simulink model "Controller_with_3DOF_model"  (R2020a)
settings: Solver=ode4  StartTime=0.0  StopTime=130  FixedStep=0.04  RelTol=1e-3
values from neighbouring files (symbols this model uses):
  a = L*(1-WF)    (= 1.81178)    [parameters.m]
  avg_dist = mean(dist_array)    [parameters.m]
  b = L*WF    (= 1.32822)    [parameters.m]
  c2r = 1*(pi/180)    (= 0.0174532925199)    [parameters.m]
  m = 2257    [parameters.m]
  n = 12    [parameters.m]
  X_waypoints = [699934.396313 699934.399288 699934.40266 699934.406729 699934.412322 699934.420718 699934.432825 699934.447764 699934.466045 699934.489064 699934.518829 699934.556022 ... (1891 elements, 1x1891)]    [reference_path.mat]
  Y_waypoints = [-5195211.87 -5195211.87121 -5195211.87256 -5195211.87411 -5195211.87621 -5195211.87926 -5195211.88371 -5195211.88919 -5195211.8959 -5195211.90452 -5195211.91606 -5195211.93042 ... (1891 elements, 1x1891)]    [reference_path.mat]
  Yaw_waypoint = [130.3891316 130.393107092 130.397831164 130.402362614 130.409271739 130.418915142 130.433687561 130.450949982 130.469948658 130.492496199 130.52263774 130.556853638 ... (1891 elements, 1x1891)]    [reference_path.mat]
undefined symbols (not defined in the file or in its folder): C_alpha, Kp_crosstrack, Kp_yaw, Kp_yaw_rate, mass
libraries: simulink_extras x11, simulink x3, autolibshared x1
settings Model: Creator=bhagwat  LastModifiedBy=root

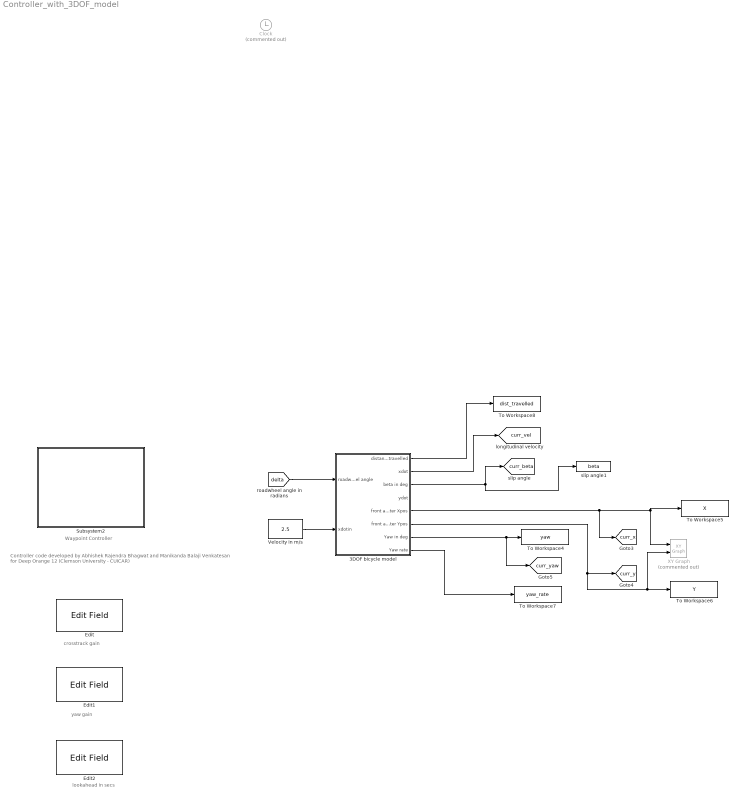
== system Controller_with_3DOF_model ==
  note: Controller code developed by Abhishek Rajendra Bhagwat and
      | Manikanda Balaji Venkatesan for Deep Orange 12 (Clemson University - CUICAR)
  note: crosstrack gain
  note: Waypoint Controller
  note: yaw gain
  note: lookahead in secs
  3DOF bicycle model : Subsystem
  Clock : Clock  Commented=on
  Edit : EditField  LabelPosition=Hide  ShowInitialText=on  Alignment=Center
  Edit1 : EditField  LabelPosition=Hide  ShowInitialText=on  Alignment=Center
  Edit2 : EditField  LabelPosition=Hide  ShowInitialText=on  Alignment=Center
  Subsystem2 : Subsystem
  To Workspace4 : ToWorkspace  VariableName=yaw  SaveFormat=Timeseries  SampleTime=-1
  To Workspace5 : ToWorkspace  VariableName=X  SampleTime=-1
  To Workspace6 : ToWorkspace  VariableName=Y  SampleTime=-1
  To Workspace7 : ToWorkspace  VariableName=yaw_rate  SaveFormat=Timeseries  SampleTime=-1
  To Workspace8 : ToWorkspace  VariableName=dist_travelled  SaveFormat=Timeseries  SampleTime=-1
  Velocity in m/s : Constant  Value=2.5
  XY Graph : simulink/Sinks/XY Graph  Commented=on  xmin=-1000  xmax=1000  ymin=-1000  ymax=1000  st=-1
  slip angle1 : ToWorkspace  VariableName=beta  SaveFormat=Timeseries  SampleTime=-1
  tag scope: curr_beta=global, curr_vel=global, curr_x=global, curr_y=global, curr_yaw=global
  wires:
  3DOF bicycle model/7(Yaw in deg) -> [curr_yaw], To Workspace4/1
  3DOF bicycle model/3(beta in deg) -> [curr_beta], slip angle1/1
  3DOF bicycle model/6(front axle center Ypos) -> XY Graph/2, To Workspace6/1, [curr_y]
  3DOF bicycle model/5(front axle center Xpos) -> To Workspace5/1, XY Graph/1, [curr_x]
  [delta] -> 3DOF bicycle model/1(roadwheel angle)
  Velocity in m/s/1 -> 3DOF bicycle model/2(xdotin)
  3DOF bicycle model/1(distance travelled) -> To Workspace8/1
  3DOF bicycle model/2(xdot) -> [curr_vel]
  3DOF bicycle model/8(Yaw rate) -> To Workspace7/1

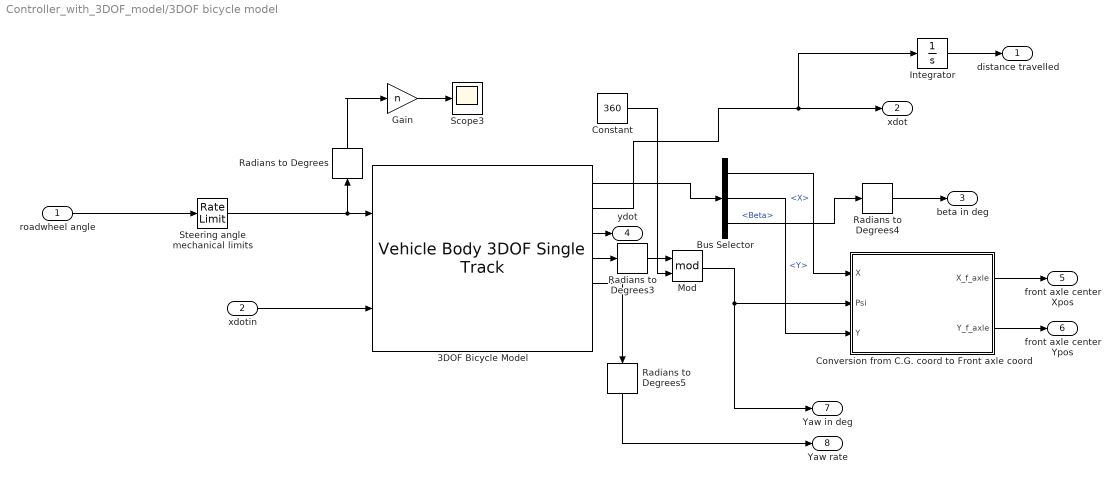
== system Controller_with_3DOF_model/3DOF bicycle model ==
  roadwheel angle : Inport
  xdotin : Inport  Port=2
  3DOF Bicycle Model : autolibshared/Vehicle Body 3DOF Single Track  trackMode=Single (bicycle)  inputMode=External longitudinal velocity  frontSteerMode=on  rearSteerMode=off  windMode=off  muMode=off  extFMode=off  extMMode=off  extXo=off  extpsio=off  extxdoto=off  extro=off  extYo=off  extTamb=off  extydoto=off  aMode=2  NF=2  NR=2  m=m  a=a  b=b  h=0.35  X_o=X_waypoints(1)  xdot_o=0  CalphaMode=off  sigmaMode=off  d=0  w=[1.4,1.4]  Cy_f=C1_0  Cy_r=C2_0  sigma_f=.1  sigma_r=.1  alpha_f_brk=[-.1 .1]  Cy_f_data=[-9e3 9e3]  alpha_r_brk=[-.1 .1]  Cy_r_data=[-9e3 9e3]  Y_o=Y_waypoints(1)  ydot_o=0  Izz=2500  psi_o=(360+100-Yaw_waypoint(1))*c2r  r_o=0  Af=2  Cd=.3  Cl=.1  Cpm=.1  beta_w=[0:0.01:0.3]  Cs=[0:0.03:0.9]  Cym=[0:0.01:0.3]  Pabs=101325  Tair=273  g=9.81  mu=1  xdot_tol=.01  Fznom=5000  Fxtire_sat=7e4  Fytire_sat=7e4  longOff=0  latOff=0  vertOff=0  wrapAng=off
      settings: SourceProductBaseCode=PW,MT,VE,VP
  Bus Selector : BusSelector  OutputSignals=InertFrm.Cg.Disp.X,InertFrm.Cg.Disp.Y,BdyFrm.Cg.Ang.Beta
  Constant : Constant  Value=360
  Conversion from C.G. coord to Front axle coord : Subsystem
  Gain : Gain  Gain=n
  Integrator : Integrator
  Mod : Math  Operator=mod  SaturateOnIntegerOverflow=on
  Radians to Degrees{,3..5} (4 alike) : simulink_extras/Transformations/Radians to Degrees
  Scope3 : Scope
  Steering angle mechanical limits : RateLimiter  RisingSlewLimit=275/n  FallingSlewLimit=-275/n  SampleTimeMode=inherited
  distance travelled : Outport
  xdot : Outport  Port=2
  beta in deg : Outport  Port=3
  ydot : Outport  Port=4
  front axle center Xpos : Outport  Port=5
  front axle center Ypos : Outport  Port=6
  Yaw in deg : Outport  Port=7
  Yaw rate : Outport  Port=8
  wires:
  3DOF Bicycle Model/3 -> ydot/1
  Steering angle mechanical limits/1 -> Radians to Degrees/1, 3DOF Bicycle Model/1
  Radians to Degrees5/1 -> Yaw rate/1
  3DOF Bicycle Model/4 -> Radians to Degrees3/1
  3DOF Bicycle Model/2 -> xdot/1, Integrator/1
  3DOF Bicycle Model/1 -> Bus Selector/1
  roadwheel angle/1 -> Steering angle mechanical limits/1
  Radians to Degrees4/1 -> beta in deg/1
  Mod/1 -> Yaw in deg/1, Conversion from C.G. coord to Front axle coord/2(Psi)
  xdotin/1 -> 3DOF Bicycle Model/2
  3DOF Bicycle Model/5 -> Radians to Degrees5/1
  Bus Selector/2 -> Conversion from C.G. coord to Front axle coord/3(Y)  "<Y>"
  Integrator/1 -> distance travelled/1
  Radians to Degrees3/1 -> Mod/1
  Bus Selector/1 -> Conversion from C.G. coord to Front axle coord/1(X)  "<X>"
  Bus Selector/3 -> Radians to Degrees4/1  "<Beta>"
  Radians to Degrees/1 -> Gain/1
  Gain/1 -> Scope3/1
  Conversion from C.G. coord to Front axle coord/2(Y_f_axle) -> front axle center Ypos/1
  Conversion from C.G. coord to Front axle coord/1(X_f_axle) -> front axle center Xpos/1
  Constant/1 -> Mod/2

== system Controller_with_3DOF_model/Subsystem2 ==
  Reference waypoints : Subsystem
  Steering Wheel Angle : Subsystem
  Vehicle state : Subsystem

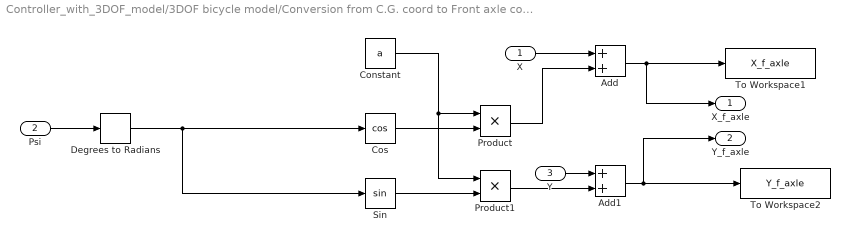
== system Controller_with_3DOF_model/3DOF bicycle model/Conversion from C.G. coord to Front axle coord ==
  X : Inport
  Psi : Inport  Port=2
  Y : Inport  Port=3
  Add : Sum
  Add1 : Sum
  Constant : Constant  Value=a
  Cos : Trigonometry  Operator=cos
  Degrees to Radians : simulink_extras/Transformations/Degrees to Radians
  Product : Product
  Product1 : Product
  Sin : Trigonometry
  To Workspace1 : ToWorkspace  VariableName=X_f_axle  SaveFormat=Timeseries  SampleTime=-1
  To Workspace2 : ToWorkspace  VariableName=Y_f_axle  SaveFormat=Timeseries  SampleTime=-1
  X_f_axle : Outport
  Y_f_axle : Outport  Port=2
  wires:
  Cos/1 -> Product/2
  Sin/1 -> Product1/2
  Product/1 -> Add/2
  Constant/1 -> Product1/1, Product/1
  X/1 -> Add/1
  Add1/1 -> Y_f_axle/1, To Workspace2/1
  Psi/1 -> Degrees to Radians/1
  Add/1 -> To Workspace1/1, X_f_axle/1
  Product1/1 -> Add1/2
  Y/1 -> Add1/1
  Degrees to Radians/1 -> Cos/1, Sin/1

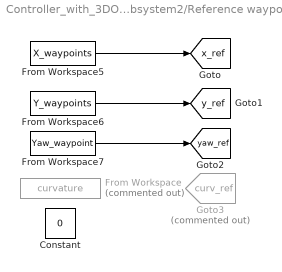
== system Controller_with_3DOF_model/Subsystem2/Reference waypoints ==
  Constant : Constant  Value=0
  From Workspace : FromWorkspace  Commented=on  VariableName=curvature
  From Workspace5 : FromWorkspace  VariableName=X_waypoints
  From Workspace6 : FromWorkspace  VariableName=Y_waypoints
  From Workspace7 : FromWorkspace  VariableName=Yaw_waypoint
  Goto3 : Goto  Commented=on  GotoTag=curv_ref  TagVisibility=global
  tag scope: x_ref=global, y_ref=global, yaw_ref=global
  wires:
  From Workspace5/1 -> [x_ref]
  From Workspace6/1 -> [y_ref]
  From Workspace7/1 -> [yaw_ref]

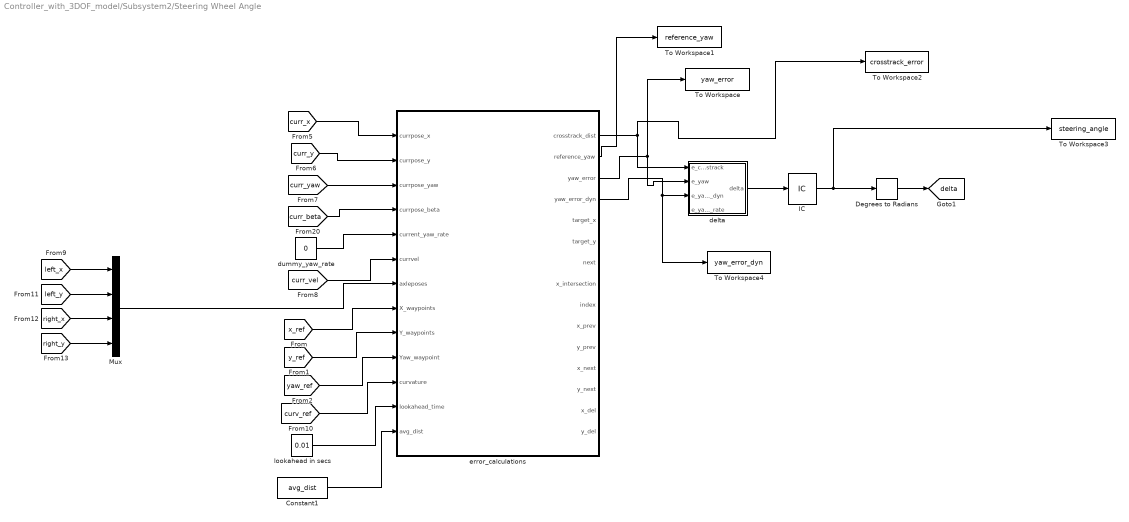
== system Controller_with_3DOF_model/Subsystem2/Steering Wheel Angle ==
  Constant1 : Constant  Value=avg_dist
  Degrees to Radians : simulink_extras/Transformations/Degrees to Radians
  IC : InitialCondition  Value=0
  Mux : Mux
  To Workspace : ToWorkspace  VariableName=yaw_error  SaveFormat=Timeseries  SampleTime=-1
  To Workspace1 : ToWorkspace  VariableName=reference_yaw  SaveFormat=Timeseries  SampleTime=-1
  To Workspace2 : ToWorkspace  VariableName=crosstrack_error  SaveFormat=Timeseries  SampleTime=-1
  To Workspace3 : ToWorkspace  VariableName=steering_angle  SaveFormat=Timeseries  SampleTime=-1
  To Workspace4 : ToWorkspace  VariableName=yaw_error_dyn  SaveFormat=Timeseries  SampleTime=-1
  delta : Subsystem
  dummy_yaw_rate : Constant  Value=0
  error_calculations : MATLAB Function  TreatAsAtomicUnit=on
  lookahead in secs : Constant  Value=0.01
  tag scope: delta=global
  wires:
  [yaw_ref] -> error_calculations/10(Yaw_waypoint)
  [curv_ref] -> error_calculations/11(curvature)
  [x_ref] -> error_calculations/8(X_waypoints)
  [y_ref] -> error_calculations/9(Y_waypoints)
  error_calculations/3(yaw_error) -> delta/2(e_yaw), To Workspace/1
  [curr_x] -> error_calculations/1(currpose_x)
  [curr_y] -> error_calculations/2(currpose_y)
  [curr_yaw] -> error_calculations/3(currpose_yaw)
  dummy_yaw_rate/1 -> error_calculations/5(current_yaw_rate)
  [curr_vel] -> error_calculations/6(currvel)
  Mux/1 -> error_calculations/7(axleposes)
  [left_x] -> Mux/1
  [left_y] -> Mux/2
  [right_x] -> Mux/3
  [right_y] -> Mux/4
  [curr_beta] -> error_calculations/4(currpose_beta)
  error_calculations/2(reference_yaw) -> To Workspace1/1
  Degrees to Radians/1 -> [delta]
  delta/1(delta) -> IC/1
  IC/1 -> To Workspace3/1, Degrees to Radians/1
  error_calculations/4(yaw_error_dyn) -> To Workspace4/1, delta/3(e_yaw_dyn)
  Constant1/1 -> error_calculations/13(avg_dist)
  lookahead in secs/1 -> error_calculations/12(lookahead_time)
  error_calculations/1(crosstrack_dist) -> To Workspace2/1, delta/1(e_crosstrack)

== system Controller_with_3DOF_model/Subsystem2/Vehicle state ==
  left_right_wheel_coordinates : Subsystem
  position : Subsystem  Commented=on

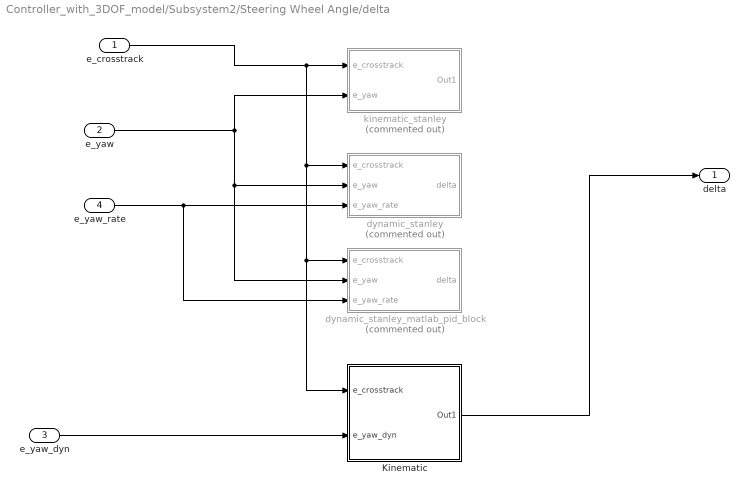
== system Controller_with_3DOF_model/Subsystem2/Steering Wheel Angle/delta ==
  e_crosstrack : Inport
  e_yaw : Inport  Port=2
  e_yaw_dyn : Inport  Port=3
  e_yaw_rate : Inport  Port=4
  Kinematic : Subsystem
  dynamic_stanley : Subsystem  Commented=on
  dynamic_stanley_matlab_pid_block : Subsystem  Commented=on
  kinematic_stanley : Subsystem  Commented=on
  delta : Outport
  wires:
  e_crosstrack/1 -> Kinematic/1(e_crosstrack), dynamic_stanley_matlab_pid_block/1(e_crosstrack), dynamic_stanley/1(e_crosstrack), kinematic_stanley/1(e_crosstrack)
  e_yaw/1 -> dynamic_stanley_matlab_pid_block/2(e_yaw), dynamic_stanley/2(e_yaw), kinematic_stanley/2(e_yaw)
  e_yaw_rate/1 -> dynamic_stanley_matlab_pid_block/3(e_yaw_rate), dynamic_stanley/3(e_yaw_rate)
  Kinematic/1(Out1) -> delta/1
  e_yaw_dyn/1 -> Kinematic/2(e_yaw_dyn)

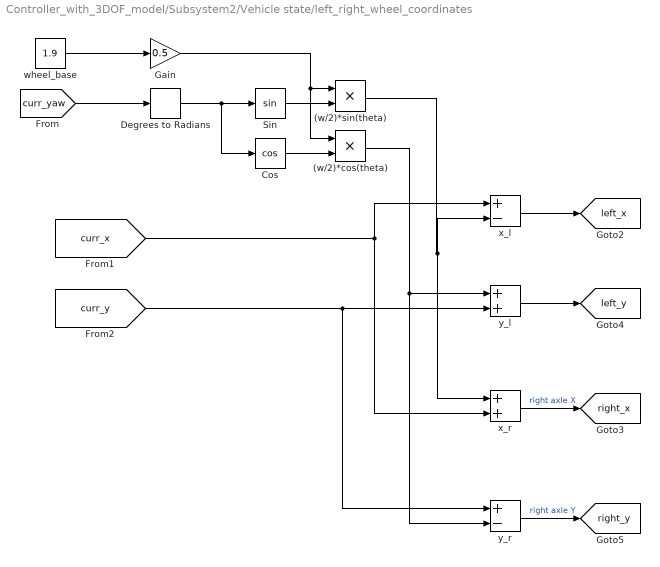
== system Controller_with_3DOF_model/Subsystem2/Vehicle state/left_right_wheel_coordinates ==
  (w/2)*cos(theta) : Product
  (w/2)*sin(theta) : Product
  Cos : Trigonometry  Operator=cos
  Degrees to Radians : simulink_extras/Transformations/Degrees to Radians
  Gain : Gain  Gain=0.5
  Sin : Trigonometry
  wheel_base : Constant  Value=1.9
  x_l : Sum  Inputs=+-
  x_r : Sum
  y_l : Sum
  y_r : Sum  Inputs=+-
  tag scope: left_x=global, left_y=global, right_x=global, right_y=global
  wires:
  wheel_base/1 -> Gain/1
  Degrees to Radians/1 -> Cos/1, Sin/1
  Sin/1 -> (w/2)*sin(theta)/2
  Gain/1 -> (w/2)*cos(theta)/1, (w/2)*sin(theta)/1
  Cos/1 -> (w/2)*cos(theta)/2
  (w/2)*sin(theta)/1 -> x_r/1, x_l/2
  [curr_y] -> y_r/1, y_l/2
  [curr_x] -> x_r/2, x_l/1
  (w/2)*cos(theta)/1 -> y_r/2, y_l/1
  [curr_yaw] -> Degrees to Radians/1
  y_r/1 -> [right_y]  "right axle Y"
  x_r/1 -> [right_x]  "right axle X"
  x_l/1 -> [left_x]
  y_l/1 -> [left_y]

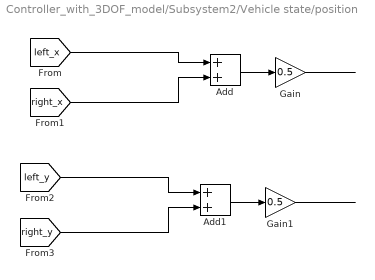
== system Controller_with_3DOF_model/Subsystem2/Vehicle state/position ==
  Add : Sum
  Add1 : Sum
  Gain : Gain  Gain=0.5
  Gain1 : Gain  Gain=0.5
  wires:
  Add/1 -> Gain/1
  Gain1/1 -> ?
  Gain/1 -> ?
  Add1/1 -> Gain1/1
  [left_x] -> Add/1
  [right_x] -> Add/2
  [left_y] -> Add1/1
  [right_y] -> Add1/2

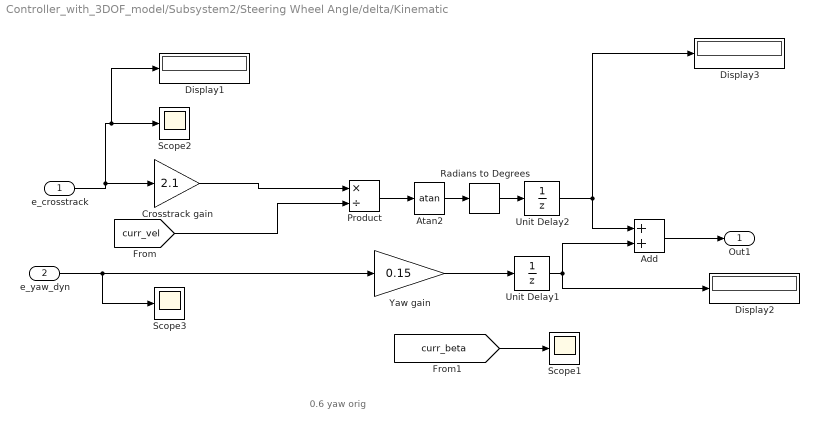
== system Controller_with_3DOF_model/Subsystem2/Steering Wheel Angle/delta/Kinematic ==
  note: 0.6 yaw orig
  e_crosstrack : Inport
  e_yaw_dyn : Inport  Port=2
  Add : Sum
  Atan2 : Trigonometry  Operator=atan  OutputSignalType=real
  Crosstrack gain : Gain  Gain=2.1
  Display1 : Display
  Display2 : Display
  Display3 : Display
  Product : Product  Inputs=*/
  Radians to Degrees : simulink_extras/Transformations/Radians to Degrees
  Scope1 : Scope
  Scope2 : Scope
  Scope3 : Scope
  Unit Delay1 : UnitDelay  SampleTime=-1  HasFrameUpgradeWarning=on
  Unit Delay2 : UnitDelay  SampleTime=-1  HasFrameUpgradeWarning=on
  Yaw gain : Gain  Gain=0.15
  Out1 : Outport
  wires:
  Add/1 -> Out1/1
  [curr_vel] -> Product/2
  Radians to Degrees/1 -> Unit Delay2/1
  Atan2/1 -> Radians to Degrees/1
  Unit Delay1/1 -> Add/2, Display2/1
  e_yaw_dyn/1 -> Scope3/1, Yaw gain/1
  Yaw gain/1 -> Unit Delay1/1
  Crosstrack gain/1 -> Product/1
  Product/1 -> Atan2/1
  e_crosstrack/1 -> Display1/1, Scope2/1, Crosstrack gain/1
  [curr_beta] -> Scope1/1
  Unit Delay2/1 -> Display3/1, Add/1

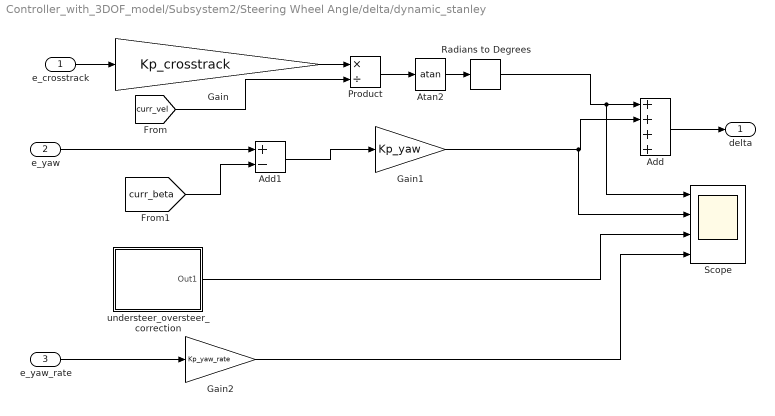
== system Controller_with_3DOF_model/Subsystem2/Steering Wheel Angle/delta/dynamic_stanley ==
  e_crosstrack : Inport
  e_yaw : Inport  Port=2
  e_yaw_rate : Inport  Port=3
  Add : Sum  Inputs=++++
  Add1 : Sum  Inputs=+-
  Atan2 : Trigonometry  Operator=atan  OutputSignalType=real
  Gain : Gain  Gain=Kp_crosstrack
  Gain1 : Gain  Gain=Kp_yaw
  Gain2 : Gain  Gain=Kp_yaw_rate
  Product : Product  Inputs=*/
  Radians to Degrees : simulink_extras/Transformations/Radians to Degrees
  Scope : Scope  NumInputPorts=4
  understeer_oversteer_correction : Subsystem
  delta : Outport
  wires:
  e_crosstrack/1 -> Gain/1
  Product/1 -> Atan2/1
  Gain/1 -> Product/1
  e_yaw/1 -> Add1/1
  Gain1/1 -> Scope/2, Add/2
  Atan2/1 -> Radians to Degrees/1
  Radians to Degrees/1 -> Scope/1, Add/1
  [curr_vel] -> Product/2
  Add/1 -> delta/1
  [curr_beta] -> Add1/2
  Add1/1 -> Gain1/1
  understeer_oversteer_correction/1(Out1) -> Scope/3
  e_yaw_rate/1 -> Gain2/1
  Gain2/1 -> Scope/4

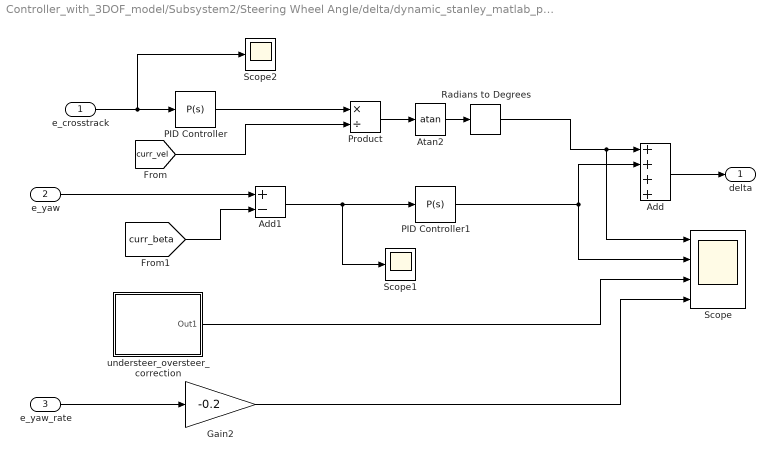
== system Controller_with_3DOF_model/Subsystem2/Steering Wheel Angle/delta/dynamic_stanley_matlab_pid_block ==
  e_crosstrack : Inport
  e_yaw : Inport  Port=2
  e_yaw_rate : Inport  Port=3
  Add : Sum  Inputs=++++
  Add1 : Sum  Inputs=+-
  Atan2 : Trigonometry  Operator=atan  OutputSignalType=real
  Gain2 : Gain  Gain=-0.2
  PID Controller : simulink/Continuous/PID Controller  Controller=P  Form=Parallel  TimeDomain=Continuous-time  UseExternalTs=off  SampleTime=-1  IntegratorMethod=Forward Euler  FilterMethod=Forward Euler  ControllerParametersSource=internal  P=2  I=-1  D=0  UseFilter=on  N=100  TunerSelectOption=Transfer Function Based (PID Tuner App)  InitialConditionSource=internal  InitialConditionForIntegrator=0  InitialConditionForFilter=0  DifferentiatorICPrevScaledInput=0  ExternalReset=none  TrackingMode=off  Kt=1  LimitOutput=off  UpperSaturationLimit=inf  LowerSaturationLimit=-inf  LinearizeAsGain=on  AntiWindupMode=none  Kb=1  POutMin=[]  POutMax=[]  IOutMin=[]  IOutMax=[]  DOutMin=[]  DOutMax=[]  NOutMin=[]  NOutMax=[]  SumOutMin=[]  SumOutMax=[]  SaturationOutMin=[]  SaturationOutMax=[]  PParamMin=[]  PParamMax=[]  IParamMin=[]  IParamMax=[]  DParamMin=[]  DParamMax=[]  NParamMin=[]  NParamMax=[]  KbParamMin=[]  KbParamMax=[]  KtParamMin=[]  KtParamMax=[]  KbOutMin=[]  KbOutMax=[]  KtOutMin=[]  KtOutMax=[]  IntegratorOutMin=[]  IntegratorOutMax=[]  FilterOutMin=[]  FilterOutMax=[]  SumI1OutMin=[]  SumI1OutMax=[]  SumI2OutMin=[]  SumI2OutMax=[]  SumI3OutMin=[]  SumI3OutMax=[]  SumI4OutMin=[]  SumI4OutMax=[]  SumDOutMin=[]  SumDOutMax=[]  DifferentiatorOutMin=[]  DifferentiatorOutMax=[]  FilterDiffOutCoefMin=[]  FilterDiffOutCoefMax=[]  ReciprocalOutMin=[]  ReciprocalOutMax=[]  SumDenOutMin=[]  SumDenOutMax=[]  SumNumOutMin=[]  SumNumOutMax=[]  DivideOutMin=[]  DivideOutMax=[]  UdiffTsProdOutMin=[]  UdiffTsProdOutMax=[]  NTsProdOutMin=[]  NTsProdOutMax=[]  UintegralTsProdOutMin=[]  UintegralTsProdOutMax=[]  UngainTsProdOutMin=[]  UngainTsProdOutMax=[]  IntegratorContinuousStateAttributes=''  IntegratorStateMustResolveToSignalObject=off  IntegratorRTWStateStorageClass=Auto  FilterContinuousStateAttributes=''  FilterStateMustResolveToSignalObject=off  FilterRTWStateStorageClass=Auto  ParallelPVariant=InternalParameters  IdealPVariant=Disabled  IVariant=Disabled  DVariant=Disabled  IntegratorVariant=Disabled  SatVariant=Disabled  AWVariant=Disabled  PCopyVariant=Disabled  TRVariant=Disabled  FdbkBlocksVariant=Forward  IdealPFdbkVariant=Disabled  SatFdbkVariant=Disabled  DerivativeFilterVariant=Disabled  NVariant=Disabled  NCopyVariant=Disabled_SignalSpec  FilterICVariant=Disabled  IntegratorICVariant=Disabled  ExternalResetVariant=Disabled  TRSumVariant=Passthrough  SumFdbkVariant=Disabled  SumVariant=Passthrough_P  TsampFilterVariant=InternalTs  TsampNgainVariant=Passthrough  TsampIntegralVariant=Disabled_SignalSpec
  PID Controller1 : simulink/Continuous/PID Controller  Controller=P  Form=Parallel  TimeDomain=Continuous-time  UseExternalTs=off  SampleTime=-1  IntegratorMethod=Forward Euler  FilterMethod=Forward Euler  ControllerParametersSource=internal  P=0.3  I=-1  D=0  UseFilter=on  N=100  TunerSelectOption=Transfer Function Based (PID Tuner App)  InitialConditionSource=internal  InitialConditionForIntegrator=0  InitialConditionForFilter=0  DifferentiatorICPrevScaledInput=0  ExternalReset=none  TrackingMode=off  Kt=1  LimitOutput=off  UpperSaturationLimit=inf  LowerSaturationLimit=-inf  LinearizeAsGain=on  AntiWindupMode=none  Kb=1  POutMin=[]  POutMax=[]  IOutMin=[]  IOutMax=[]  DOutMin=[]  DOutMax=[]  NOutMin=[]  NOutMax=[]  SumOutMin=[]  SumOutMax=[]  SaturationOutMin=[]  SaturationOutMax=[]  PParamMin=[]  PParamMax=[]  IParamMin=[]  IParamMax=[]  DParamMin=[]  DParamMax=[]  NParamMin=[]  NParamMax=[]  KbParamMin=[]  KbParamMax=[]  KtParamMin=[]  KtParamMax=[]  KbOutMin=[]  KbOutMax=[]  KtOutMin=[]  KtOutMax=[]  IntegratorOutMin=[]  IntegratorOutMax=[]  FilterOutMin=[]  FilterOutMax=[]  SumI1OutMin=[]  SumI1OutMax=[]  SumI2OutMin=[]  SumI2OutMax=[]  SumI3OutMin=[]  SumI3OutMax=[]  SumI4OutMin=[]  SumI4OutMax=[]  SumDOutMin=[]  SumDOutMax=[]  DifferentiatorOutMin=[]  DifferentiatorOutMax=[]  FilterDiffOutCoefMin=[]  FilterDiffOutCoefMax=[]  ReciprocalOutMin=[]  ReciprocalOutMax=[]  SumDenOutMin=[]  SumDenOutMax=[]  SumNumOutMin=[]  SumNumOutMax=[]  DivideOutMin=[]  DivideOutMax=[]  UdiffTsProdOutMin=[]  UdiffTsProdOutMax=[]  NTsProdOutMin=[]  NTsProdOutMax=[]  UintegralTsProdOutMin=[]  UintegralTsProdOutMax=[]  UngainTsProdOutMin=[]  UngainTsProdOutMax=[]  IntegratorContinuousStateAttributes=''  IntegratorStateMustResolveToSignalObject=off  IntegratorRTWStateStorageClass=Auto  FilterContinuousStateAttributes=''  FilterStateMustResolveToSignalObject=off  FilterRTWStateStorageClass=Auto  ParallelPVariant=InternalParameters  IdealPVariant=Disabled  IVariant=Disabled  DVariant=Disabled  IntegratorVariant=Disabled  SatVariant=Disabled  AWVariant=Disabled  PCopyVariant=Disabled  TRVariant=Disabled  FdbkBlocksVariant=Forward  IdealPFdbkVariant=Disabled  SatFdbkVariant=Disabled  DerivativeFilterVariant=Disabled  NVariant=Disabled  NCopyVariant=Disabled_SignalSpec  FilterICVariant=Disabled  IntegratorICVariant=Disabled  ExternalResetVariant=Disabled  TRSumVariant=Passthrough  SumFdbkVariant=Disabled  SumVariant=Passthrough_P  TsampFilterVariant=InternalTs  TsampNgainVariant=Passthrough  TsampIntegralVariant=Disabled_SignalSpec
  Product : Product  Inputs=*/
  Radians to Degrees : simulink_extras/Transformations/Radians to Degrees
  Scope : Scope  NumInputPorts=4
  Scope1 : Scope
  Scope2 : Scope
  understeer_oversteer_correction : Subsystem
  delta : Outport
  wires:
  Gain2/1 -> Scope/4
  e_yaw_rate/1 -> Gain2/1
  understeer_oversteer_correction/1(Out1) -> Scope/3
  Add1/1 -> Scope1/1, PID Controller1/1
  [curr_beta] -> Add1/2
  Add/1 -> delta/1
  [curr_vel] -> Product/2
  Radians to Degrees/1 -> Add/1, Scope/1
  Atan2/1 -> Radians to Degrees/1
  PID Controller1/1 -> Add/2, Scope/2
  e_yaw/1 -> Add1/1
  PID Controller/1 -> Product/1
  Product/1 -> Atan2/1
  e_crosstrack/1 -> Scope2/1, PID Controller/1

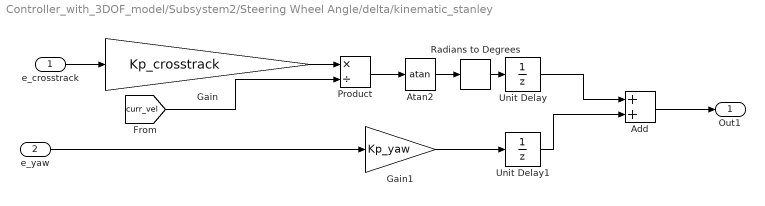
== system Controller_with_3DOF_model/Subsystem2/Steering Wheel Angle/delta/kinematic_stanley ==
  e_crosstrack : Inport
  e_yaw : Inport  Port=2
  Add : Sum
  Atan2 : Trigonometry  Operator=atan  OutputSignalType=real
  Gain : Gain  Gain=Kp_crosstrack
  Gain1 : Gain  Gain=Kp_yaw
  Product : Product  Inputs=*/
  Radians to Degrees : simulink_extras/Transformations/Radians to Degrees
  Unit Delay : UnitDelay  SampleTime=-1  HasFrameUpgradeWarning=on
  Unit Delay1 : UnitDelay  SampleTime=-1  HasFrameUpgradeWarning=on
  Out1 : Outport
  wires:
  e_crosstrack/1 -> Gain/1
  Product/1 -> Atan2/1
  Gain/1 -> Product/1
  Radians to Degrees/1 -> Unit Delay/1
  Gain1/1 -> Unit Delay1/1
  e_yaw/1 -> Gain1/1
  Unit Delay1/1 -> Add/2
  Atan2/1 -> Radians to Degrees/1
  Unit Delay/1 -> Add/1
  [curr_vel] -> Product/2
  Add/1 -> Out1/1

== system Controller_with_3DOF_model/Subsystem2/Steering Wheel Angle/delta/dynamic_stanley/understeer_oversteer_correction ==
  Gain2 : Gain  Gain=mass/( 2 * C_alpha * ( 1 + a/b))
  Product1 : Product
  Out1 : Outport
  wires:
  [curr_vel] -> Product1/1
  Gain2/1 -> Out1/1
  [yaw_rate_ref] -> Product1/2
  Product1/1 -> Gain2/1

== system Controller_with_3DOF_model/Subsystem2/Steering Wheel Angle/delta/dynamic_stanley_matlab_pid_block/understeer_oversteer_correction ==
  Gain2 : Gain  Gain=mass/( 2 * C_alpha * ( 1 + a/b))
  Product1 : Product
  Out1 : Outport
  wires:
  Product1/1 -> Gain2/1
  [yaw_rate_ref] -> Product1/2
  Gain2/1 -> Out1/1
  [curr_vel] -> Product1/1

== matlab function Controller_with_3DOF_model/Subsystem2/Steering Wheel Angle/error_calculations ==
  data: currpose_x input; crosstrack_dist output; reference_yaw output; yaw_error output; yaw_error_dyn output; target_x output; target_y output; next output; x_intersection output; currpose_y input; currpose_yaw input; currpose_beta input; current_yaw_rate input; currvel input; axleposes input; X_waypoints input; Y_waypoints input; Yaw_waypoint input; curvature input; index output; lookahead_time input; avg_dist input; x_prev output; y_prev output; x_next output; y_next output; x_del output; y_del output
%Waypoint controller code developed by Manikanda Balaji Venkatesan and
%Abhishek Bhagwat for Deep Orange 12 (Clemson University International Center for Automotive Research)

function [crosstrack_dist,reference_yaw,yaw_error,yaw_error_dyn, target_x, target_y, next,x_intersection,index,x_prev, y_prev, x_next, y_next, x_del, y_del] = fcn(currpose_x,currpose_y,currpose_yaw,currpose_beta,current_yaw_rate,currvel, axleposes, X_waypoints, Y_waypoints, Yaw_waypoint, curvature, lookahead_time, avg_dist)


%identification of closest point
no_of_waypoints = length(X_waypoints);
i = no_of_waypoints;
distance_from_current = ones(1, i);  %initialization of array used for storing the distance between current point and all waypoints
while i>0
    distance_from_current(i) = distance(currpose_x, currpose_y, X_waypoints(i), Y_waypoints(i));
    i = i - 1;
end

[~,index] = min(distance_from_current); %finding the closest waypoint as least distance point

lookahead_dist = lookahead_time*currvel; %lookahead in m for corresponding time
lookahead = lookahead_dist/avg_dist;
lookahead = round(lookahead);

%index for waypoints
% next = index+10;                   %next waypoint the vehicle should go for
next = index+0;                   %next waypoint the vehicle should go for
if next < 2
    next = 2;
end
prev = next - 1;                %previous waypoint the vehicle has crossed

target_x = X_waypoints(next);
target_y = Y_waypoints(next);

x_prev = X_waypoints(prev);
y_prev = Y_waypoints(prev);
x_next = X_waypoints(next);
y_next = Y_waypoints(next);
%poi - point of intersection
[x_intersection, y_intersection,m1,m2, x_del, y_del] = poi(currpose_x,currpose_y, x_prev, y_prev, x_next, y_next);
dist_from_next = distance(x_intersection, y_intersection, x_next, y_next);
dist_from_prev = distance(x_intersection, y_intersection, x_prev, y_prev);
dist_btw_waypoints = distance(x_prev,y_prev,x_next,y_next);


ratio = dist_from_prev/dist_btw_waypoints;
%ratio = 1 - (dist_from_next / dist_btw_waypoints); %how much vehicle has moved from last point to next point
yaw_prev = Yaw_waypoint(prev);
yaw_next = Yaw_waypoint(next);

curvature_prev = 0;
curvature_next = 0;


%yaw error calculation
% reference_yaw = yaw_prev + (yaw_next - yaw_prev) * ratio;
% reference_yaw = atan2((Y_waypoints(next)-currpose_y),(X_waypoints(next)-currpose_x));
% reference_yaw = reference_yaw*(180/pi);
% ref_bef_corr = reference_yaw;
% if (reference_yaw < -10)
%      reference_yaw = 360 + reference_yaw;
% end
% 
% yaw_error = reference_yaw - currpose_yaw;
% yaw_error_dyn = reference_yaw - (currpose_yaw + currpose_beta);
% 
% yaw_error_dyn_before = yaw_error_dyn;
% if yaw_error_dyn > 300
%     yaw_error_dyn = yaw_error_dyn - 360;
% end

%yaw error calculation
reference_yaw = yaw_prev + (yaw_next - yaw_prev) * ratio;
reference_yaw = 360-reference_yaw;
reference_yaw = mod(reference_yaw,360);
yaw_error = reference_yaw - currpose_yaw;
yaw_error_dyn = reference_yaw - currpose_yaw;
if yaw_error_dyn > 250
    yaw_error_dyn = yaw_error_dyn - 360;
end

%yaw rate error calculation
% reference_curvature = curvature_prev + (curvature_next - curvature_prev) * ratio;
% reference_yaw_rate = currvel * reference_curvature * 180 / 3.14; %yaw rate in deg/s
% yaw_rate_error = reference_yaw_rate - current_yaw_rate;


%cross track error calculation
crosstrack_dist = distance(currpose_x, currpose_y, x_intersection, y_intersection);
%cross track error sign determination
left_axle_pos = [axleposes(1), axleposes(2)];
right_axle_pos = [axleposes(3), axleposes(4)];
left_axle_dist = distance(left_axle_pos(1), left_axle_pos(2), target_x, target_y);
right_axle_dist = distance(right_axle_pos(1), right_axle_pos(2), target_x, target_y);


if left_axle_dist>right_axle_dist
    sign_path = -1;  %turning right
else
    sign_path = 1;  %turning left
end
crosstrack_dist = sign_path * crosstrack_dist;

end

function dist = distance(x1,y1,x2,y2)
dist = sqrt( (x2-x1)^2 + (y2-y1)^2 );
end

function [x_intersection, y_intersection,m1,m2,x_del, y_del] = poi(currpose_x,currpose_y, x_prev, y_prev, x_next, y_next)
    
    %equation of waypoint line is x*m1 + c1 = y
    y_del = (y_next - y_prev);
    x_del = (x_next - x_prev);
    m1 = (y_del)/(x_del);

    c1 = y_next - ( m1*x_next);
     
    %following is equation of line between current location to nearest point on waypoint path
    m2 = -1/m1;
    c2 = currpose_y - (m2*currpose_x);
    %equation of above line is m2*x + c2 = y
    
    %point of intersection of above lines
    if m1 == inf || m1 == -inf
        y_intersection = currpose_y;
        x_intersection = x_prev;
    elseif m1 == 0
        y_intersection = y_prev ;
        x_intersection = currpose_x;
    else
        y_intersection = (m1*c2 - m2*c1)/(m1 - m2);
        x_intersection = (y_intersection - c1) / m1;
    end
    
end
